simulink model "IP_LQG_PCI6221_2015a"  (R2015a)
settings: Solver=ode3  StartTime=0.0  StopTime=200  RelTol=1e-3
values from neighbouring files (symbols this model uses):
  A = [0 0 0 0 0 1 -0.0174048595758 0 -0.0173759205618 -232.025201375 0 20.7861247087 ... (25 elements, 5x5)]    [Integrator_Result.mat]    (also in Q_100_0_10_0_0__R_0d001____0d2pp____noInt.mat; Q_100_0_1_0_0__R_0d001____0d05____noInt.mat; Q_100_0_1_0_0__R_0d001____0d2pp____alpha1.mat; Q_100_0_1_0_0__R_0d001____0d2pp____alpha1___beta100.mat)
  ALPHA_MAX = 1.57079632679    [Integrator_Result.mat]    (also in Q_100_0_10_0_0__R_0d001____0d2pp____noInt.mat; Q_100_0_1_0_0__R_0d001____0d05____noInt.mat; Q_100_0_1_0_0__R_0d001____0d2pp____alpha1.mat; Q_100_0_1_0_0__R_0d001____0d2pp____alpha1___beta100.mat)
  B = [0 0 0 0 333.33674813]    [Integrator_Result.mat]    (also in Q_100_0_10_0_0__R_0d001____0d2pp____noInt.mat; Q_100_0_1_0_0__R_0d001____0d05____noInt.mat; Q_100_0_1_0_0__R_0d001____0d2pp____alpha1.mat; Q_100_0_1_0_0__R_0d001____0d2pp____alpha1___beta100.mat)
  BETA_MAX = 0.261799387799    [Integrator_Result.mat]    (also in Q_100_0_10_0_0__R_0d001____0d2pp____noInt.mat; Q_100_0_1_0_0__R_0d001____0d05____noInt.mat; Q_100_0_1_0_0__R_0d001____0d2pp____alpha1.mat; Q_100_0_1_0_0__R_0d001____0d2pp____alpha1___beta100.mat)
  C = [1  0  0  0  0; 0  0  1  0  0]    [Integrator_Result.mat]    (also in Q_100_0_10_0_0__R_0d001____0d2pp____noInt.mat; Q_100_0_1_0_0__R_0d001____0d05____noInt.mat; Q_100_0_1_0_0__R_0d001____0d2pp____alpha1.mat; Q_100_0_1_0_0__R_0d001____0d2pp____alpha1___beta100.mat)
  K = [-99.9999999929 -34.4803462076 248.902916401 37.4638671809 0.212521025017]    [Integrator_Result.mat]    (also in Q_100_0_10_0_0__R_0d001____0d2pp____noInt.mat = [-316.22776594 -103.533802305 724.463830461 109.132925574 0.; Q_100_0_1_0_0__R_0d001____0d05____noInt.mat = [-316.227765861 -102.594372714 711.33329858 108.084823842 0.; Q_100_0_1_0_0__R_0d001____0d2pp____alpha1.mat = [-316.227765861 -102.594372714 711.33329858 108.084823842 0.; Q_100_0_1_0_0__R_0d001____0d2pp____alpha1___beta100.mat = [-99.9999999916 -34.210789658 244.985138447 37.1447338159 0.)
  L = [316.229260948  0.0153881424831; 0.472858273025  20.5476858398; 0.0153881424831  1000.14458234; -0.291137577833  144.592911266; -0.14634723893  -2.7003340726]    [Integrator_Result.mat]    (also in Q_100_0_10_0_0__R_0d001____0d2pp____noInt.mat = [3.26664981927  1.13709483629; 0.981992854244  11.8725297148; Q_100_0_1_0_0__R_0d001____0d05____noInt.mat = [3.26664981927  1.13709483629; 0.981992854244  11.8725297148; Q_100_0_1_0_0__R_0d001____0d2pp____alpha1.mat = [3.26664981927  1.13709483629; 0.981992854244  11.8725297148; Q_100_0_1_0_0__R_0d001____0d2pp____alpha1___beta100.mat = [3.26664981927  1.13709483629; 0.981992854244  11.8725297148)
  TIME_DELAY = 6    [Integrator_Result.mat]    (also in Q_100_0_10_0_0__R_0d001____0d2pp____noInt.mat; Q_100_0_1_0_0__R_0d001____0d05____noInt.mat; Q_100_0_1_0_0__R_0d001____0d2pp____alpha1.mat; Q_100_0_1_0_0__R_0d001____0d2pp____alpha1___beta100.mat)
  Ts = 0.001    [Integrator_Result.mat]    (also in Q_100_0_10_0_0__R_0d001____0d2pp____noInt.mat; Q_100_0_1_0_0__R_0d001____0d05____noInt.mat; Q_100_0_1_0_0__R_0d001____0d2pp____alpha1.mat; Q_100_0_1_0_0__R_0d001____0d2pp____alpha1___beta100.mat)
  V_MAX = 5    [Integrator_Result.mat]    (also in Q_100_0_10_0_0__R_0d001____0d2pp____noInt.mat; Q_100_0_1_0_0__R_0d001____0d05____noInt.mat; Q_100_0_1_0_0__R_0d001____0d2pp____alpha1.mat; Q_100_0_1_0_0__R_0d001____0d2pp____alpha1___beta100.mat)
  V_MIN = -5    [Integrator_Result.mat]    (also in Q_100_0_10_0_0__R_0d001____0d2pp____noInt.mat; Q_100_0_1_0_0__R_0d001____0d05____noInt.mat; Q_100_0_1_0_0__R_0d001____0d2pp____alpha1.mat; Q_100_0_1_0_0__R_0d001____0d2pp____alpha1___beta100.mat)
undefined symbols (not defined in the file or in its folder): National_Instruments, PCI
libraries: sldrtlib x3, simulink x2
settings Model: SimulationMode=external  ExtModeTrigDuration=100000  Creator=Alunos  LastModifiedBy=afons
settings HardwareCC: ProdBitPerLong=64  ProdBitPerPointer=64  ProdIntDivRoundTo=Zero  ProdEndianess=LittleEndian  ProdWordSize=64  ProdHWDeviceType=Intel->x86-64  TargetBitPerLong=64  TargetBitPerPointer=64  TargetIntDivRoundTo=Zero  TargetEndianess=LittleEndian  TargetWordSize=64  TargetHWDeviceType=Intel->x86-64
settings RTWCC: SystemTargetFile=rtwin.tlc  TemplateMakefile=rtwin.tmf  Description=Simulink Desktop Real-Time  RTWCompilerOptimization=on
settings CodeAppCC: MaxIdLength=95
settings RTWinTargetCC: TargetPreCompLibLocation=C:\Program Files\MATLAB\R2015a\toolbox\sldrt\lib\win64

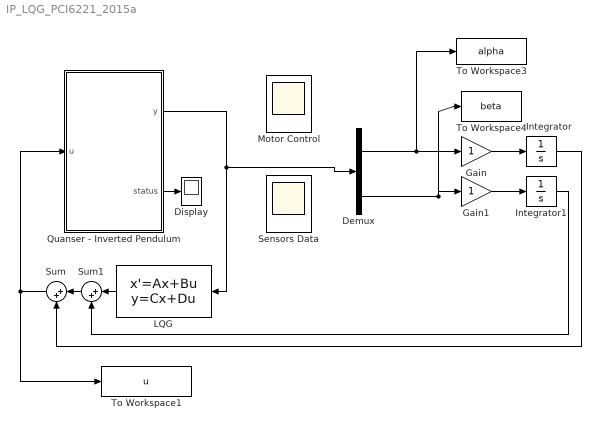
== system IP_LQG_PCI6221_2015a ==
  Demux : Demux  Outputs=2
  Display : Display
  Gain : Gain
  Gain1 : Gain
  Integrator : Integrator
  Integrator1 : Integrator
  LQG : StateSpace  A=A-B*K-L*C  B=L  C=-K  D=zeros(1,2)  X0=0
  Motor Control : Scope
      settings: Floating=on  ShowLegends=on  SaveName=ScopeData2
  Quanser - Inverted Pendulum : Subsystem
      mask Display: image('IP_QUANSER.jpg');
  Sensors Data : Scope
      settings: Floating=on  ShowLegends=on  YMin=-3.191592653589793  YMax=3.191592653589793
  Sum : Sum  Inputs=|++
  Sum1 : Sum  Inputs=|++
  To Workspace1 : ToWorkspace  VariableName=u  SampleTime=-1
  To Workspace3 : ToWorkspace  VariableName=alpha  SampleTime=-1
  To Workspace4 : ToWorkspace  VariableName=beta  SampleTime=-1
  wires:
  Quanser - Inverted Pendulum/1(y) -> LQG/1, Demux/1
  Sum/1 -> To Workspace1/1, Quanser - Inverted Pendulum/1(u)
  Quanser - Inverted Pendulum/2(status) -> Display/1
  Demux/1 -> To Workspace3/1, Gain/1
  Gain/1 -> Integrator/1
  Integrator1/1 -> Sum1/2
  Demux/2 -> To Workspace4/1, Gain1/1
  Gain1/1 -> Integrator1/1
  LQG/1 -> Sum1/1
  Integrator/1 -> Sum/2
  Sum1/1 -> Sum/1

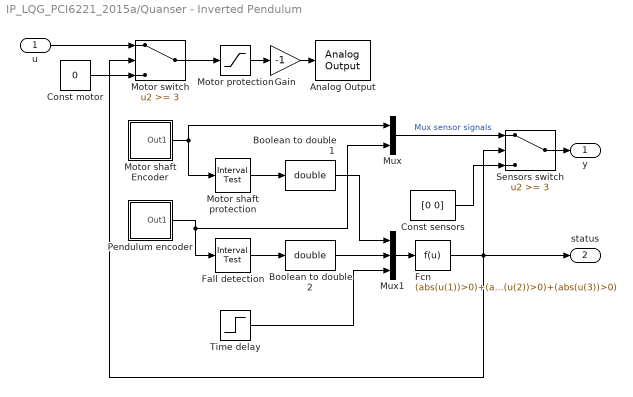
== system IP_LQG_PCI6221_2015a/Quanser - Inverted Pendulum ==
  u : Inport
  Analog Output : sldrtlib/Analog Output  SampleTime=Ts  MaxMissedTicks=10  ShowMissedTicks=off  YieldWhenWaiting=off  DrvName=National_Instruments/PCI-6221  DrvAddress=4294967295  DrvOptions=[0 0 0 2 2]  Channels=1  RangeMode=1  VoltRange=1  InitialValue=0  FinalValue=0
      settings: AttributesFormatString=National Instruments\nPCI-6221 [auto]
  Boolean to double 1 : DataTypeConversion  OutDataTypeStr=double
  Boolean to double 2 : DataTypeConversion  OutDataTypeStr=double
  Const motor : Constant  Value=0
  Const sensors : Constant  Value=[0 0]
  Fall detection : simulink/Logic and Bit Operations/Interval Test  IntervalClosedRight=on  uplimit=BETA_MAX  IntervalClosedLeft=on  lowlimit=-BETA_MAX  OutDataTypeStr=uint8
  Fcn : Fcn  Expr=(abs(u(1))>0)+(abs(u(2))>0)+(abs(u(3))>0)
  Gain : Gain  Gain=-1
  Motor protection : Saturate  UpperLimit=V_MAX  LowerLimit=V_MIN
  Motor shaft Encoder : Subsystem
  Motor shaft protection : simulink/Logic and Bit Operations/Interval Test  IntervalClosedRight=on  uplimit=ALPHA_MAX  IntervalClosedLeft=on  lowlimit=-ALPHA_MAX  OutDataTypeStr=uint8
  Motor switch : Switch  Threshold=3
  Mux : Mux  Inputs=2
  Mux1 : Mux  Inputs=3
  Pendulum encoder : Subsystem
  Sensors switch : Switch  Threshold=3
  Time delay : Step  Time=TIME_DELAY  SampleTime=0
  y : Outport
  status : Outport  Port=2
  wires:
  u/1 -> Motor switch/1
  Motor switch/1 -> Motor protection/1
  Const motor/1 -> Motor switch/3
  Motor shaft Encoder/1(Out1) -> Mux/1, Motor shaft protection/1
  Pendulum encoder/1(Out1) -> Fall detection/1, Mux/2
  Mux1/1 -> Fcn/1
  Fcn/1 -> Sensors switch/2, status/1, Motor switch/2
  Time delay/1 -> Mux1/3
  Fall detection/1 -> Boolean to double 2/1
  Boolean to double 2/1 -> Mux1/2
  Motor shaft protection/1 -> Boolean to double 1/1
  Boolean to double 1/1 -> Mux1/1
  Const sensors/1 -> Sensors switch/3
  Mux/1 -> Sensors switch/1  "Mux sensor signals"
  Sensors switch/1 -> y/1
  Gain/1 -> Analog Output/1
  Motor protection/1 -> Gain/1

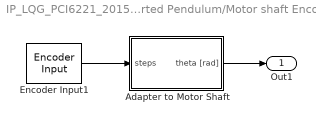
== system IP_LQG_PCI6221_2015a/Quanser - Inverted Pendulum/Motor shaft Encoder ==
  Adapter to Motor Shaft : Subsystem
  Encoder Input1 : sldrtlib/Encoder Input  SampleTime=Ts  MaxMissedTicks=inf  ShowMissedTicks=off  YieldWhenWaiting=off  DrvName=National_Instruments/PCI-6221  DrvAddress=4294967295  DrvOptions=[0 0 0 2 2]  Channels=1  QuadMode=3  IndexPulse=2  InputFilter=Inf  DataType=1
      settings: AttributesFormatString=National Instruments\nPCI-6221 [auto]
  Out1 : Outport
  wires:
  Encoder Input1/1 -> Adapter to Motor Shaft/1(steps)
  Adapter to Motor Shaft/1(theta [rad]) -> Out1/1

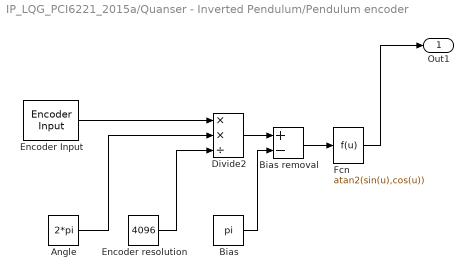
== system IP_LQG_PCI6221_2015a/Quanser - Inverted Pendulum/Pendulum encoder ==
  Angle : Constant  Value=2*pi
  Bias : Constant  Value=pi
  Bias removal : Sum  Inputs=+-
  Divide2 : Product  Inputs=**/
  Encoder resolution : Constant  Value=4096
  Encoder Input : sldrtlib/Encoder Input  SampleTime=Ts  MaxMissedTicks=inf  ShowMissedTicks=off  YieldWhenWaiting=off  DrvName=National_Instruments/PCI-6221  DrvAddress=4294967295  DrvOptions=[0 0 0 2 2]  Channels=2  QuadMode=3  IndexPulse=2  InputFilter=Inf  DataType=1
      settings: AttributesFormatString=National Instruments\nPCI-6221 [auto]
  Fcn : Fcn  Expr=atan2(sin(u),cos(u))
  Out1 : Outport
  wires:
  Bias/1 -> Bias removal/2
  Encoder resolution/1 -> Divide2/3
  Divide2/1 -> Bias removal/1
  Fcn/1 -> Out1/1
  Encoder Input/1 -> Divide2/1
  Bias removal/1 -> Fcn/1
  Angle/1 -> Divide2/2

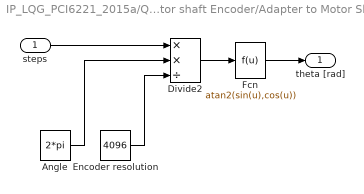
== system IP_LQG_PCI6221_2015a/Quanser - Inverted Pendulum/Motor shaft Encoder/Adapter to Motor Shaft ==
  steps : Inport
  Angle : Constant  Value=2*pi
  Divide2 : Product  Inputs=**/
  Encoder resolution : Constant  Value=4096
  Fcn : Fcn  Expr=atan2(sin(u),cos(u))
  theta [rad] : Outport
  wires:
  Angle/1 -> Divide2/2
  Encoder resolution/1 -> Divide2/3
  steps/1 -> Divide2/1
  Divide2/1 -> Fcn/1
  Fcn/1 -> theta [rad]/1
